simulink model "LightingSystem_v2"  (R2022a)
settings: Solver=VariableStepAuto  StartTime=0.0  StopTime=10.0  RelTol=1e-3
libraries: simulink x2
settings Model: Creator=AAMIR  LastModifiedBy=AAMIR

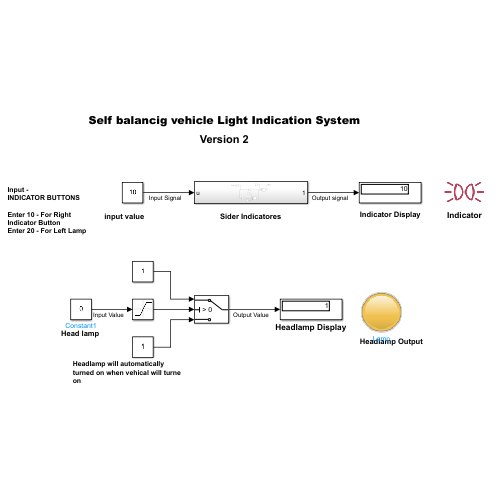
[thumbnail: Simulink's stored preview of the top-level diagram]
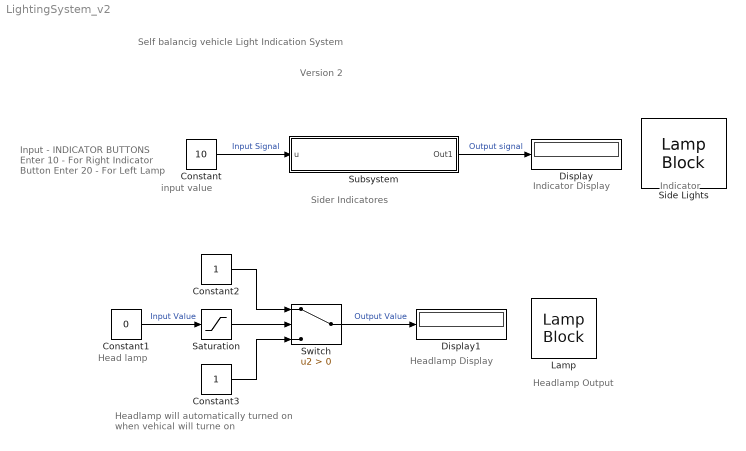
== system LightingSystem_v2 ==
  note: Indicator
  note: Headlamp Output
  note: Headlamp will automatically turned on when vehical will turne on
  note: Headlamp Display
  note: Head lamp
  note: input value
  note: Version 2
  note: Self balancig vehicle Light Indication System
  note: Sider Indicatores
  note: Input -
      | INDICATOR BUTTONS
      |
      | Enter 10 - For Right Indicator Button
      | Enter 20 - For Left Lamp
  note: Indicator Display
  Constant : Constant  Value=10
  Constant1 : Constant  Value=0
  Constant2 : Constant
  Constant3 : Constant
  Display : Display
  Display1 : Display
  Lamp : LampBlock  LabelPosition=Hide
  Saturation : Saturate  UpperLimit=1  LowerLimit=0
  Side Lights : LampBlock  LabelPosition=Hide  Icon=SideLights
  Subsystem : Subsystem
  Switch : Switch  Criteria=u2 > Threshold  SaturateOnIntegerOverflow=off  InputSameDT=off
  wires:
  Constant/1 -> Subsystem/1(u)  "Input Signal"
  Subsystem/1(Out1) -> Display/1  "Output signal"
  Constant1/1 -> Saturation/1  "Input Value"
  Saturation/1 -> Switch/2
  Constant2/1 -> Switch/1
  Constant3/1 -> Switch/3
  Switch/1 -> Display1/1  "Output Value"

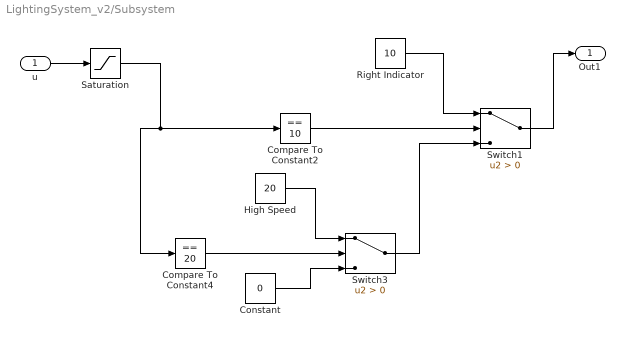
== system LightingSystem_v2/Subsystem ==
  u : Inport
  Compare To Constant2 : simulink/Logic and Bit Operations/Compare To Constant  relop===  const=10  OutDataTypeStr=boolean
  Compare To Constant4 : simulink/Logic and Bit Operations/Compare To Constant  relop===  const=20  OutDataTypeStr=boolean
  Constant : Constant  Value=0
  High Speed : Constant  Value=20
  Right Indicator : Constant  Value=10
  Saturation : Saturate  UpperLimit=20  LowerLimit=0
  Switch1 : Switch  Criteria=u2 > Threshold  SaturateOnIntegerOverflow=off  InputSameDT=off
  Switch3 : Switch  Criteria=u2 > Threshold  SaturateOnIntegerOverflow=off  InputSameDT=off
  Out1 : Outport
  wires:
  Compare To Constant2/1 -> Switch1/2
  u/1 -> Saturation/1
  Compare To Constant4/1 -> Switch3/2
  Switch3/1 -> Switch1/3
  Right Indicator/1 -> Switch1/1
  High Speed/1 -> Switch3/1
  Constant/1 -> Switch3/3
  Switch1/1 -> Out1/1
  Saturation/1 -> Compare To Constant4/1, Compare To Constant2/1
